simulink model "PIC_MOTOR_FOR_CALIBRATION"  (R2016a)
settings: Solver=ode23s  StartTime=0.0  StopTime=10  FixedStep=0.001  RelTol=1e-5
undefined symbols (not defined in the file): b, I, Ka, Ke, L, R
settings Model: Creator=bhorton  LastModifiedBy=bhorton
settings DataIOCC: SaveOutput=off  SignalLogging=off  DSMLogging=off  VisualizeSimOutput=off  SaveTime=off
settings DebuggingCC: AlgebraicLoopMsg=error  AllowSymbolicDim=off
settings ModelReferenceCC: PropagateSignalLabelsOutOfModel=off
settings GRTTargetCC: GeneratePreprocessorConditionals=Use local settings

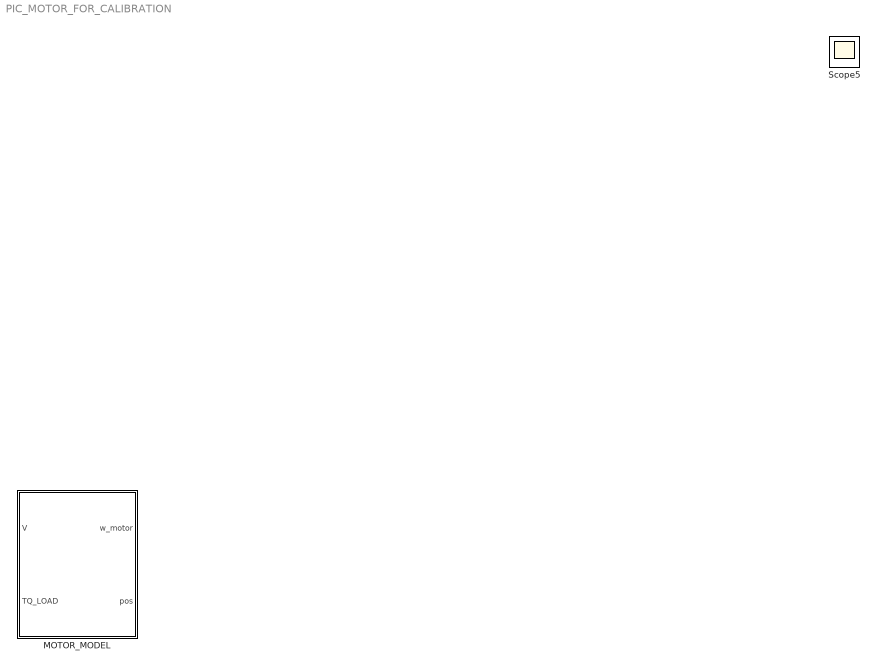
== system PIC_MOTOR_FOR_CALIBRATION ==
  MOTOR_MODEL : Subsystem  mask(DC motor){K=Ka, B=b, J=I, GearRatio=1, R=R, L=L, Kb=Ke, ID=0}
      mask prompts: K "Torque constant (N.m/A)"; B "Viscous friction co-efficient (N.m.s)"; J "Rotor Inertia (kg.m^2)"; GearRatio "Gear ratio (w_motor/w_wheel)"; R "Armature resistance (ohms)"; L "Armature Inductance (Henry)"; Kb "Back Emf constant (V.sec/rad)"; ID "Motor_ID  (#1 to #4)"
      mask help: DC motor
      mask Display: disp('DC motor')
  Scope5 : Scope
  wires:
  ? -> ?

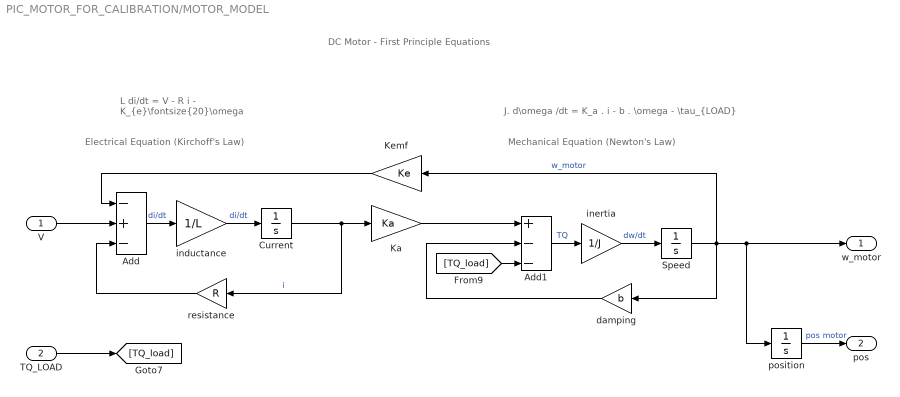
== system PIC_MOTOR_FOR_CALIBRATION/MOTOR_MODEL ==
  note: Electrical Equation
      | (Kirchoff's Law)
  note: DC Motor - First Principle Equations
  note: J. d\omega /dt = K_a . i - b . \omega - \tau_{LOAD}
  note: L di/dt = V - R i - K_{e}\fontsize{20}\omega
  note: Mechanical Equation
      | (Newton's Law)
  V : Inport
  TQ_LOAD : Inport  Port=2
  Add : Sum  Inputs=-+-
  Add1 : Sum  Inputs=+--
  Current : Integrator
  Ka : Gain  Gain=Ka
  Kemf : Gain  Gain=Ke
  Speed : Integrator
  damping : Gain  Gain=b
  inductance : Gain  Gain=1/L
  inertia : Gain  Gain=1/J
  position : Integrator
  resistance : Gain  Gain=R
  w_motor : Outport
  pos : Outport  Port=2
  wires:
  V/1 -> Add/2
  [TQ_load] -> Add1/3
  TQ_LOAD/1 -> [TQ_load]
  position/1 -> pos/1  "pos motor"
  Kemf/1 -> Add/1
  resistance/1 -> Add/3
  Add/1 -> inductance/1  "di/dt"
  Current/1 -> resistance/1, Ka/1  "i"
  Add1/1 -> inertia/1  "TQ"
  Speed/1 -> damping/1, w_motor/1, position/1, Kemf/1  "w_motor"
  inductance/1 -> Current/1  "di/dt"
  Ka/1 -> Add1/1
  damping/1 -> Add1/2
  inertia/1 -> Speed/1  "dw/dt"
